simulink model "lab7"  (R2018b)
settings: Solver=ode4  StartTime=0.0  StopTime=20.0  FixedStep=0.01  RelTol=1e-3
values from neighbouring files (symbols this model uses):
  A = [-4, -4, 0; 1, 0 ,0; 0, 1, 0]    [scriptlab2.m]    (also in scriptlab3.m = [-1, 0, 0; -1, -2 ,-101; 1, 1, 0]; scriptlab5.m = [0 , 0, 0; 1, 0 , -1; 0,1,2]; scriptlab7.m = [0,0,0;1,0,-1;0,1,2])
  Ac = double(Ac)    [scriptlab4.m]    (also in scriptlab7.m = J + H*F*M)
  B = [1;0;0]    [scriptlab2.m]    (also in scriptlab3.m = [0,1;1,-1;0,0]; scriptlab5.m = [0,-1;1,0;0,1]; scriptlab7.m = [0,-1;1,0;0,1])
  Bc = double(Bc)    [scriptlab4.m]    (also in scriptlab7.m = K + H*F*N)
  C = [0,1,2]    [scriptlab2.m]    (also in scriptlab3.m = [1,0,101]; scriptlab5.m = [1,0,1]; scriptlab7.m = [1,0,1])
  D = 0    [scriptlab2.m]    (also in scriptlab3.m = [0,0]; scriptlab7.m = [0, 0])
  Fc = F*M    [scriptlab7.m]
  Gc = F*N    [scriptlab7.m]
settings Model: Creator=grecu  LastModifiedBy=grecu

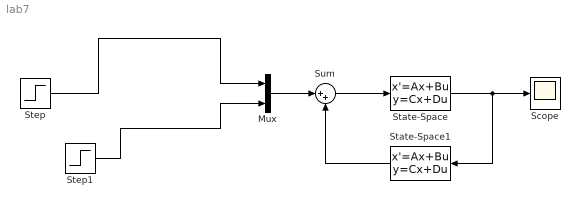
== system lab7 ==
  Mux : Mux  Inputs=2
  Scope : Scope
  State-Space : StateSpace  A=A  B=B  C=C  D=D  InitialCondition=0
  State-Space1 : StateSpace  A=Ac  B=Bc  C=Fc  D=Gc  InitialCondition=0
  Step : Step  SampleTime=0
  Step1 : Step  After=-2  SampleTime=0
  Sum : Sum  Inputs=|++
  wires:
  Mux/1 -> Sum/1
  Step/1 -> Mux/1
  Step1/1 -> Mux/2
  Sum/1 -> State-Space/1
  State-Space1/1 -> Sum/2
  State-Space/1 -> State-Space1/1, Scope/1
